simulink model "Gradient_DREM"  (R2025b)
settings: Solver=ode23tb  StartTime=0.0  StopTime=50  FixedStep=0.01  MaxStep=1e-3  RelTol=1e-3
settings Model: Creator=sasha  LastModifiedBy=Stealth
settings SolverCC: AlgebraicLoopSolver=TrustRegion
settings RTWCC: GPUComputeCapability=3.5

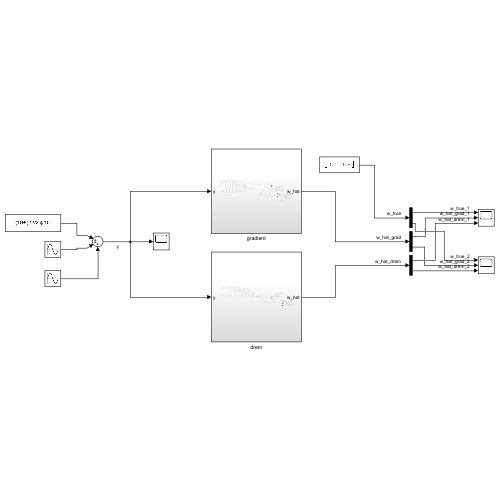
[thumbnail: Simulink's stored preview of the top-level diagram]
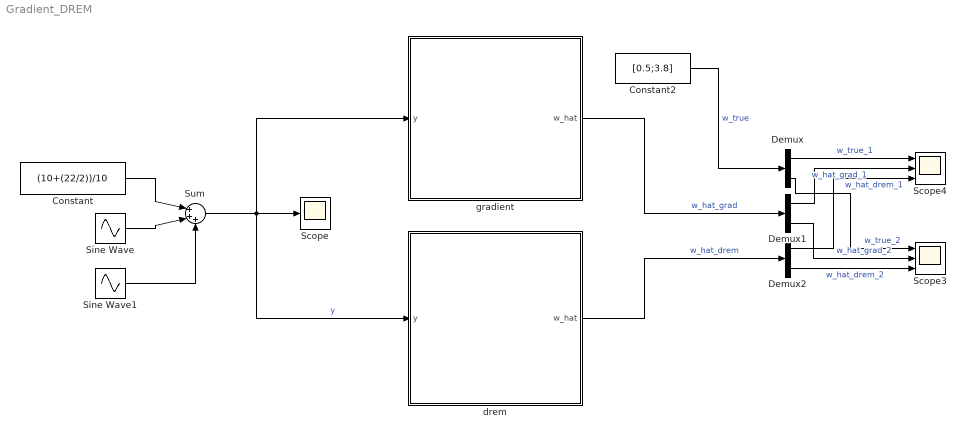
== system Gradient_DREM ==
  Constant : Constant  Value=(10+(22/2))/10
  Constant2 : Constant  Value=[0.5;3.8]
  Demux : Demux  Outputs=2
  Demux1 : Demux  Outputs=2
  Demux2 : Demux  Outputs=2
  Scope : Scope
      settings: ActiveDisplayYMinimum=-5.94936  ActiveDisplayYMaximum=11.54937
  Scope3 : Scope  NumInputPorts=3
      settings: ActiveDisplayYMinimum=-1.3593548868386089  ActiveDisplayYMaximum=5.0060994061301436
  Scope4 : Scope  NumInputPorts=3
      settings: ActiveDisplayYMinimum=0.34532  ActiveDisplayYMaximum=1.89144  DataLoggingVariableName=ScopeData2
  Sine Wave : Sin  Amplitude=2+1  Frequency=(2+10)/2  Phase=pi*(1/(100-22))  SampleTime=0
  Sine Wave1 : Sin  Amplitude=2  Frequency=(2-4)^2+2.1  Phase=pi+(pi*(1/(100-22))*2)  SampleTime=0
  Sum : Sum  Inputs=|+++
  drem : Subsystem
  gradient : Subsystem
  wires:
  Constant/1 -> Sum/1
  Sine Wave/1 -> Sum/2
  Sine Wave1/1 -> Sum/3
  Sum/1 -> Scope/1, gradient/1(y), drem/1(y)  "y"
  Constant2/1 -> Demux/1  "w_true"
  drem/1(w_hat) -> Demux2/1  "w_hat_drem"
  gradient/1(w_hat) -> Demux1/1  "w_hat_grad"
  Demux/1 -> Scope4/1  "w_true_1"
  Demux1/1 -> Scope4/2  "w_hat_grad_1"
  Demux2/2 -> Scope3/3  "w_hat_drem_2"
  Demux/2 -> Scope3/1  "w_true_2"
  Demux2/1 -> Scope4/3  "w_hat_drem_1"
  Demux1/2 -> Scope3/2  "w_hat_grad_2"

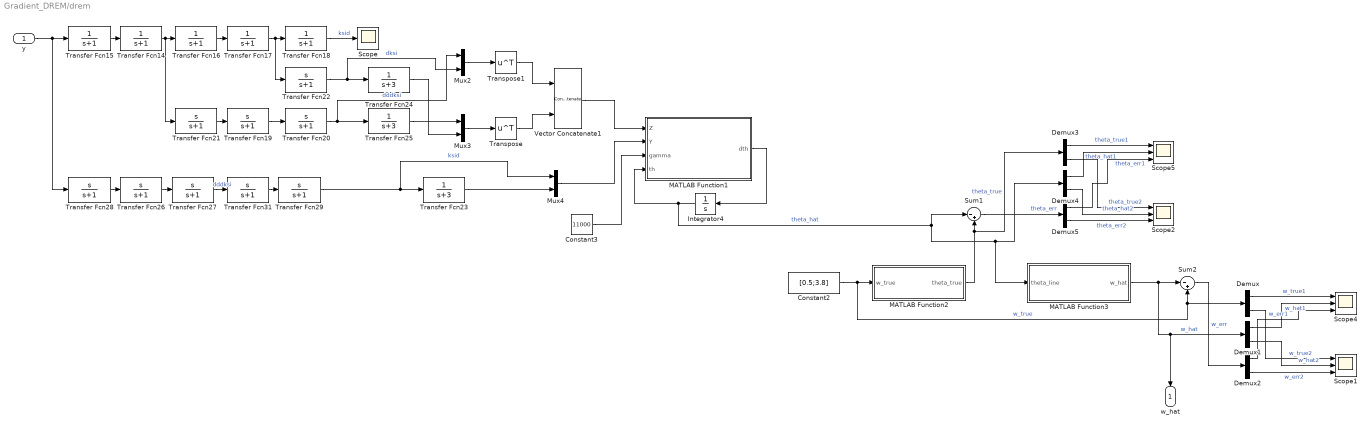
== system Gradient_DREM/drem ==
  y : Inport
  Constant2 : Constant  Value=[0.5;3.8]
  Constant3 : Constant  Value=11000
  Demux{,1..5} (6 alike) : Demux  Outputs=2
  Integrator4 : Integrator  InitialCondition=[0;0]
  MATLAB Function1 : MATLAB Function  TreatAsAtomicUnit=on
  MATLAB Function2 : MATLAB Function  TreatAsAtomicUnit=on
  MATLAB Function3 : MATLAB Function  TreatAsAtomicUnit=on
  Mux2 : Mux  Inputs=2
  Mux3 : Mux  Inputs=2
  Mux4 : Mux  Inputs=2
  Scope : Scope
  Scope{1..2,4..5} (4 alike) : Scope  NumInputPorts=3
      Scope1 settings: ActiveDisplayYMinimum=-0.475  ActiveDisplayYMaximum=4.275  DataLoggingVariableName=ScopeData4
      Scope2 settings: ActiveDisplayYMinimum=-3.5526133156575206  ActiveDisplayYMaximum=1.6689734439366219  DataLoggingVariableName=ScopeData5
      Scope4 settings: ActiveDisplayYMinimum=-0.3009722077922079  ActiveDisplayYMaximum=0.69834012987012994  DataLoggingVariableName=ScopeData3
      Scope5 settings: ActiveDisplayYMinimum=-25.80576  ActiveDisplayYMaximum=11.11576  DataLoggingVariableName=ScopeData6
  Sum1 : Sum  Inputs=|-+
  Sum2 : Sum  Inputs=|-+
  Transfer Fcn{14..18} (5 alike) : TransferFcn  Denominator=[1 1]
  Transfer Fcn{19..22,26..29,31} (9 alike) : TransferFcn  Numerator=[1 0]  Denominator=[1 1]
  Transfer Fcn23 : TransferFcn  Denominator=[1 3]
  Transfer Fcn24 : TransferFcn  Denominator=[1 3]
  Transfer Fcn25 : TransferFcn  Denominator=[1 3]
  Transpose : Math  Operator=transpose
  Transpose1 : Math  Operator=transpose
  Vector Concatenate1 : Concatenate  Mode=Multidimensional array
  w_hat : Outport
  wires:
  Mux4/1 -> MATLAB Function1/2(Y)
  Transfer Fcn26/1 -> Transfer Fcn27/1
  Transfer Fcn14/1 -> Transfer Fcn21/1, Transfer Fcn16/1
  Transfer Fcn16/1 -> Transfer Fcn17/1
  Transpose/1 -> Vector Concatenate1/2
  Transfer Fcn28/1 -> Transfer Fcn26/1
  Mux2/1 -> Transpose1/1
  Transfer Fcn25/1 -> Mux3/1
  Transfer Fcn23/1 -> Mux4/2
  Vector Concatenate1/1 -> MATLAB Function1/1(Z)
  Transfer Fcn17/1 -> Transfer Fcn22/1, Transfer Fcn18/1
  Mux3/1 -> Transpose/1
  MATLAB Function1/1(dth) -> Integrator4/1
  Transfer Fcn20/1 -> Mux2/1, Transfer Fcn25/1  "dddksi"
  Transfer Fcn24/1 -> Mux3/2
  Transfer Fcn29/1 -> Mux4/1, Transfer Fcn23/1  "ksid"
  Transfer Fcn21/1 -> Transfer Fcn19/1
  Transfer Fcn22/1 -> Transfer Fcn24/1, Mux2/2  "dksi"
  Transfer Fcn31/1 -> Transfer Fcn29/1
  Transfer Fcn19/1 -> Transfer Fcn20/1
  Transfer Fcn27/1 -> Transfer Fcn31/1  "dddksi"
  Constant3/1 -> MATLAB Function1/3(gamma)
  Transfer Fcn15/1 -> Transfer Fcn14/1
  Transpose1/1 -> Vector Concatenate1/1
  Transfer Fcn18/1 -> Scope/1  "ksid"
  MATLAB Function3/1(w_hat) -> w_hat/1, Demux1/1, Sum2/1  "w_hat"
  Sum2/1 -> Demux2/1  "w_err"
  Constant2/1 -> Sum2/2, Demux/1, MATLAB Function2/1(w_true)  "w_true"
  Sum1/1 -> Demux5/1  "theta_err"
  MATLAB Function2/1(theta_true) -> Demux3/1, Sum1/2  "theta_true"
  Integrator4/1 -> Sum1/1, Demux4/1, MATLAB Function3/1(theta_line), MATLAB Function1/4(th)  "theta_hat"
  y/1 -> Transfer Fcn28/1, Transfer Fcn15/1
  Demux/1 -> Scope4/1  "w_true1"
  Demux1/1 -> Scope4/2  "w_hat1"
  Demux2/1 -> Scope4/3  "w_err1"
  Demux/2 -> Scope1/1  "w_true2"
  Demux1/2 -> Scope1/2  "w_hat2"
  Demux2/2 -> Scope1/3  "w_err2"
  Demux4/1 -> Scope5/2  "theta_hat1"
  Demux4/2 -> Scope2/2  "theta_hat2"
  Demux3/2 -> Scope2/1  "theta_true2"
  Demux5/1 -> Scope5/3  "theta_err1"
  Demux3/1 -> Scope5/1  "theta_true1"
  Demux5/2 -> Scope2/3  "theta_err2"

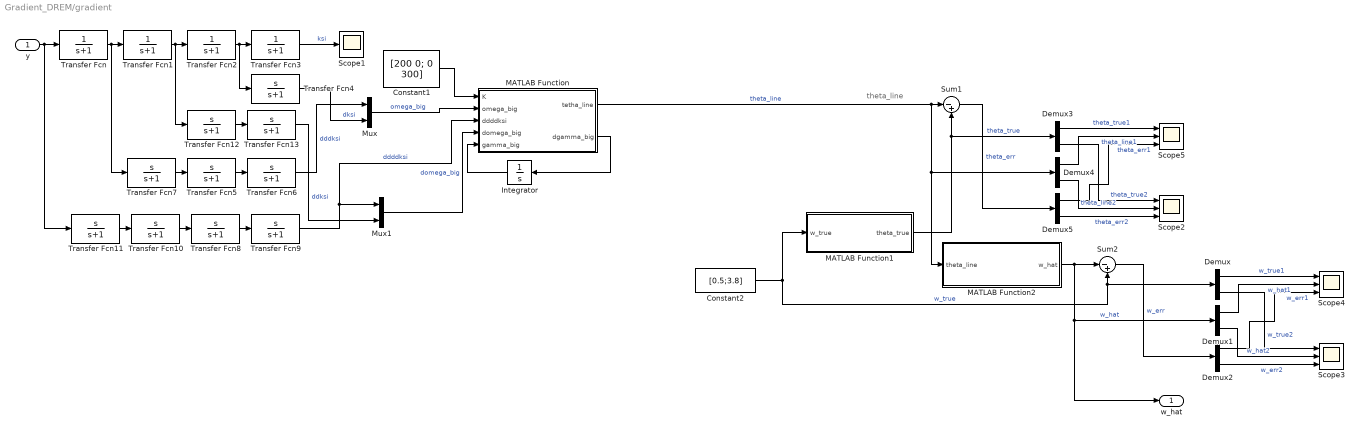
== system Gradient_DREM/gradient ==
  note: theta_line
  y : Inport
  Constant1 : Constant  Value=[200 0; 0 300]
  Constant2 : Constant  Value=[0.5;3.8]
  Demux{,1..5} (6 alike) : Demux  Outputs=2
  Integrator : Integrator  IgnoreLimit=on
  MATLAB Function : MATLAB Function  TreatAsAtomicUnit=on
  MATLAB Function1 : MATLAB Function  TreatAsAtomicUnit=on
  MATLAB Function2 : MATLAB Function  TreatAsAtomicUnit=on
  Mux : Mux  Inputs=2
  Mux1 : Mux  Inputs=2
  Scope1 : Scope
      settings: ActiveDisplayYMinimum=-0.38676  ActiveDisplayYMaximum=3.48083  DataLoggingVariableName=ScopeData2
  Scope{2..5} (4 alike) : Scope  NumInputPorts=3
      Scope2 settings: ActiveDisplayYMinimum=-11.97829  ActiveDisplayYMaximum=8.36829  DataLoggingVariableName=ScopeData8
      Scope3 settings: ActiveDisplayYMinimum=-1.8527  ActiveDisplayYMaximum=5.6527  DataLoggingVariableName=ScopeData2
      Scope4 settings: ActiveDisplayYMinimum=-1.60928  ActiveDisplayYMaximum=2.10928  DataLoggingVariableName=ScopeData7
      Scope5 settings: ActiveDisplayYMinimum=-28.20472  ActiveDisplayYMaximum=13.51472  DataLoggingVariableName=ScopeData9
  Sum1 : Sum  Inputs=|-+
  Sum2 : Sum  Inputs=|-+
  Transfer Fcn{,1..3} (4 alike) : TransferFcn  Denominator=[1 1]
  Transfer Fcn{4..13} (10 alike) : TransferFcn  Numerator=[1 0]  Denominator=[1 1]
  w_hat : Outport
  wires:
  Mux/1 -> MATLAB Function/2(omega_big)  "omega_big"
  MATLAB Function/1(tetha_line) -> Demux4/1, MATLAB Function2/1(theta_line), Sum1/1  "theta_line"
  Transfer Fcn10/1 -> Transfer Fcn8/1
  Transfer Fcn8/1 -> Transfer Fcn9/1
  Transfer Fcn9/1 -> MATLAB Function/3(ddddksi), Mux1/1  "ddddksi"
  Transfer Fcn12/1 -> Transfer Fcn13/1
  y/1 -> Transfer Fcn11/1, Transfer Fcn/1
  Transfer Fcn7/1 -> Transfer Fcn5/1
  Transfer Fcn/1 -> Transfer Fcn7/1, Transfer Fcn1/1
  MATLAB Function/2(dgamma_big) -> Integrator/1
  Integrator/1 -> MATLAB Function/5(gamma_big)
  Transfer Fcn4/1 -> Mux/2  "dksi"
  Constant1/1 -> MATLAB Function/1(K)
  Transfer Fcn11/1 -> Transfer Fcn10/1
  Mux1/1 -> MATLAB Function/4(domega_big)  "domega_big"
  Transfer Fcn5/1 -> Transfer Fcn6/1
  Transfer Fcn6/1 -> Mux/1  "dddksi"
  Transfer Fcn2/1 -> Transfer Fcn4/1, Transfer Fcn3/1
  Transfer Fcn13/1 -> Mux1/2  "ddksi"
  Transfer Fcn1/1 -> Transfer Fcn12/1, Transfer Fcn2/1
  Transfer Fcn3/1 -> Scope1/1  "ksi"
  Sum1/1 -> Demux5/1  "theta_err"
  Constant2/1 -> Demux/1, Sum2/2, MATLAB Function1/1(w_true)  "w_true"
  MATLAB Function1/1(theta_true) -> Demux3/1, Sum1/2  "theta_true"
  MATLAB Function2/1(w_hat) -> Demux1/1, w_hat/1, Sum2/1  "w_hat"
  Sum2/1 -> Demux2/1  "w_err"
  Demux1/1 -> Scope4/2  "w_hat1"
  Demux1/2 -> Scope3/2  "w_hat2"
  Demux/2 -> Scope3/1  "w_true2"
  Demux2/1 -> Scope4/3  "w_err1"
  Demux/1 -> Scope4/1  "w_true1"
  Demux2/2 -> Scope3/3  "w_err2"
  Demux4/1 -> Scope5/2  "theta_line1"
  Demux4/2 -> Scope2/2  "theta_line2"
  Demux3/2 -> Scope2/1  "theta_true2"
  Demux5/1 -> Scope5/3  "theta_err1"
  Demux3/1 -> Scope5/1  "theta_true1"
  Demux5/2 -> Scope2/3  "theta_err2"

== matlab function Gradient_DREM/drem/MATLAB Function1 ==
  data: Z input; Y input; gamma input; th input; dth output
function dth  = fcn(Z,Y, gamma, th)
[s1, s2] = size(Z);
adjZ = zeros(size(Z));
p = 1:s1;

for i = 1:s1
    for j = 1:s2
        minor = Z(setdiff(p, i), setdiff(p, j));
        adjZ(j, i) = (-1)^(i + j)*det(minor);
    end
end

delta = det(Z);
zz = adjZ*Y;
dth = gamma*delta*(zz - delta*th);

== matlab function Gradient_DREM/gradient/MATLAB Function ==
  data: K input; tetha_line output; omega_big input; ddddksi input; dgamma_big output; domega_big input; gamma_big input
function [tetha_line, dgamma_big] = fcn(K, omega_big, ddddksi, domega_big, gamma_big)

tetha_line = gamma_big + K*omega_big*ddddksi;
dgamma_big = -K*omega_big*omega_big'*tetha_line-K*domega_big*ddddksi;

== matlab function Gradient_DREM/gradient/MATLAB Function1 ==
  data: w_true input; theta_true output
function theta_true = w_to_theta_true(w_true)

theta_true = zeros(2,1);
theta_true(1) = -1 * (w_true(1)^2 + w_true(2)^2);
theta_true(2) = -1 * (w_true(1)^2) * (w_true(2)^2);

== matlab function Gradient_DREM/gradient/MATLAB Function2 ==
  data: theta_line input; w_hat output
function w_hat = theta2omega(theta_line)

S1 = -1 * theta_line(1);
S2 = -1 * theta_line(2);

D = S1^2 - 4*S2; 
if D < 0
    D = 0;
end

lam1 = 0.5*(S1 + sqrt(D));
lam2 = 0.5*(S1 - sqrt(D));

if lam1 < 0, lam1 = 0; end
if lam2 < 0, lam2 = 0; end

w1 = max(sqrt(lam1),0.5);
w2 = max(sqrt(lam2),0.5);

w_hat = [w2; w1];

== matlab function Gradient_DREM/drem/MATLAB Function2 ==
  data: w_true input; theta_true output
function theta_true = w_to_theta_true(w_true)

theta_true = zeros(2,1);
theta_true(1) = -1 * (w_true(1)^2 + w_true(2)^2);
theta_true(2) = -1 * (w_true(1)^2) * (w_true(2)^2);

== matlab function Gradient_DREM/drem/MATLAB Function3 ==
  data: theta_line input; w_hat output
function w_hat = theta2omega(theta_line)

S1 = -1 * theta_line(1);
S2 = -1 * theta_line(2);

D = S1^2 - 4*S2; 
if D < 0
    D = 0;
end

lam1 = 0.5*(S1 + sqrt(D));
lam2 = 0.5*(S1 - sqrt(D));

if lam1 < 0, lam1 = 0; end
if lam2 < 0, lam2 = 0; end

w1 = max(sqrt(lam1),0.5);
w2 = max(sqrt(lam2),0.5);

w_hat = [w2; w1];
